simulink model "pitchAndRoll"  (R2025a)
settings: Solver=FixedStepAuto  StartTime=0.0  StopTime=30  FixedStep=0.005  RelTol=1e-3
model workspace (MAT data in the model file):
  lowerLimit = 25
  speedMax = 10
  upperLimit = 75
libraries: simulink x3, simulink_extras x1
settings Model: PacingRate=0.100000  ParameterArgumentNames=speedMax  LastModifiedBy=alexc
settings SolverCC: ZeroCrossAlgorithm=Adaptive
settings OptimizationCC: BlockReduction=off  DefaultParameterBehavior=Inlined  BufferReuse=off
settings DebuggingCC: IgnoredZcDiagnostic=none
settings RTWCC: GPUComputeCapability=3.5

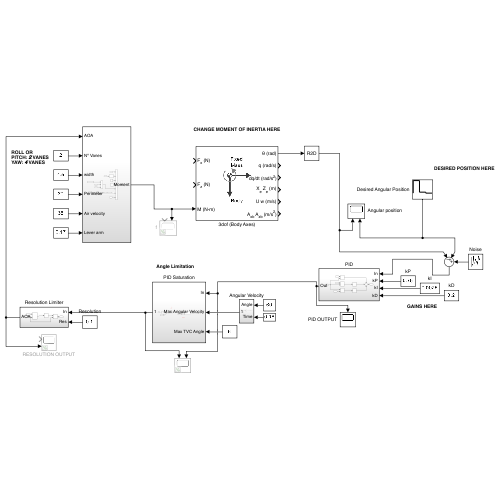
[thumbnail: Simulink's stored preview of the top-level diagram]
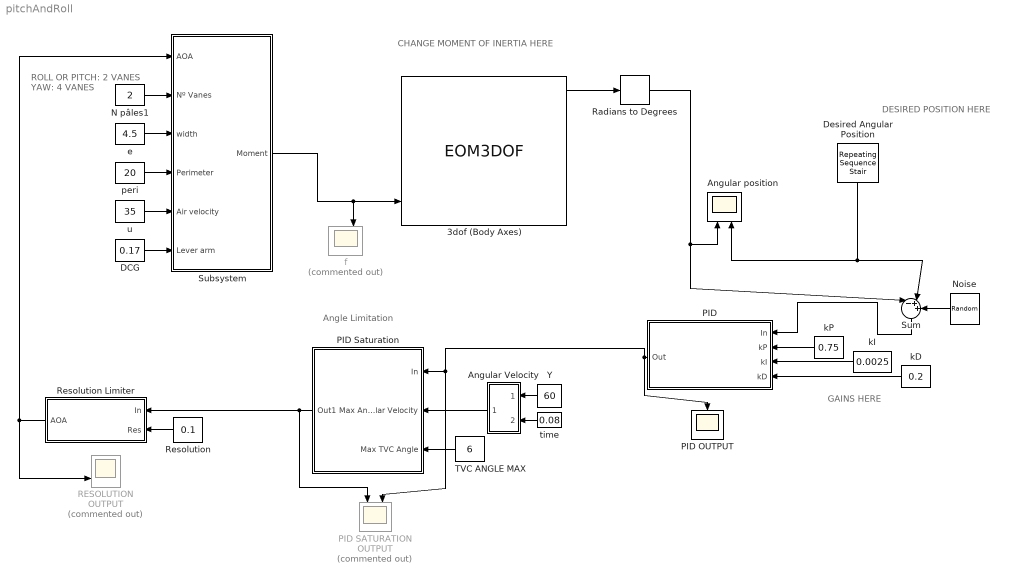
== system pitchAndRoll ==
  note: Angle Limitation
  note: GAINS HERE
  note: DESIRED POSITION HERE
  note: CHANGE MOMENT OF INERTIA HERE
  note: ROLL OR PITCH: 2 VANES
      | YAW: 4 VANES
  3dof (Body Axes) : EOM3DOF  mass=4.4  Iyy=0.045
  Angular Velocity : Subsystem
  Angular position : Scope  NumInputPorts=2
      settings: ActiveDisplayYMinimum=-1.25  ActiveDisplayYMaximum=11.25
  DCG : Constant  Value=0.17
  Desired Angular Position : simulink/Sources/Repeating Sequence Stair  OutValues=[10 2.5 2]  tsamp=1  OutMin=[]  OutMax=[]  OutDataTypeStr=double  OutputDataTypeScalingMode=double  OutDataType=fixdt(0,8)  ConRadixGroup=Best Precision: Vector-wise  OutScaling=2^-12
  N pâles1 : Constant  Value=2
  Noise : UniformRandomNumber  Minimum=-0.2  Maximum=0.2  Seed=414  SampleTime=0.02
  PID : Subsystem
  PID OUTPUT : Scope
      settings: ActiveDisplayYMinimum=-109.29716  ActiveDisplayYMaximum=117.18163  DataLoggingVariableName=ScopeData2
  PID SATURATION OUTPUT : Scope  Commented=on  NumInputPorts=2
      settings: ActiveDisplayYMinimum=-14.97719  ActiveDisplayYMaximum=15.01757  DataLoggingVariableName=ScopeData3
  PID Saturation : Subsystem
  RESOLUTION OUTPUT : Scope  Commented=on  NumInputPorts=2
      settings: ActiveDisplayYMinimum=-4.75  ActiveDisplayYMaximum=4.75
  Radians to Degrees : simulink_extras/Transformations/Radians to Degrees
  Resolution : Constant  Value=0.1
  Resolution Limiter : Subsystem
  Subsystem : Subsystem
  Sum : Sum  Inputs=|-++
  TVC ANGLE MAX : Constant  Value=6
  Y : Constant  Value=60
  e : Constant  Value=4.5
  f : Scope  Commented=on  NumInputPorts=2
      settings: ActiveDisplayYMinimum=-0.10188  ActiveDisplayYMaximum=0.10188  DataLoggingVariableName=ScopeData3
  kD : Constant  Value=0.2
  kI : Constant  Value=0.0025
  kP : Constant  Value=0.75
  peri : Constant  Value=20
  time : Constant  Value=0.08
  u : Constant  Value=35
  wires:
  Desired Angular Position/1 -> Angular position/2, Sum/2
  Radians to Degrees/1 -> Angular position/1, Sum/1
  3dof (Body Axes)/1 -> Radians to Degrees/1
  N pâles1/1 -> Subsystem/2(Nº Vanes)
  Subsystem/1(Moment) -> 3dof (Body Axes)/3, f/2
  DCG/1 -> Subsystem/6(Lever arm)
  u/1 -> Subsystem/5(Air velocity)
  e/1 -> Subsystem/3(width)
  Sum/1 -> PID/1(In)
  kP/1 -> PID/2(kP)
  kI/1 -> PID/3(kI)
  kD/1 -> PID/4(kD)
  Angular Velocity/1(Out1) -> PID Saturation/2(Max Angular Velocity)
  Y/1 -> Angular Velocity/1(Angle)
  time/1 -> Angular Velocity/2(Time)
  Resolution/1 -> Resolution Limiter/2(Res)
  PID/1(Out) -> PID OUTPUT/1, PID SATURATION OUTPUT/2, PID Saturation/1(In)
  TVC ANGLE MAX/1 -> PID Saturation/3(Max TVC Angle)
  Resolution Limiter/1(AOA) -> Subsystem/1(AOA), RESOLUTION OUTPUT/2
  PID Saturation/1(Out1) -> Resolution Limiter/1(In), PID SATURATION OUTPUT/1
  Noise/1 -> Sum/3
  peri/1 -> Subsystem/4(Perimeter)

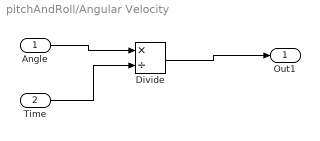
== system pitchAndRoll/Angular Velocity ==
  Angle : Inport
  Time : Inport  Port=2
  Divide : Product  Inputs=*/
  Out1 : Outport
  wires:
  Time/1 -> Divide/2
  Angle/1 -> Divide/1
  Divide/1 -> Out1/1

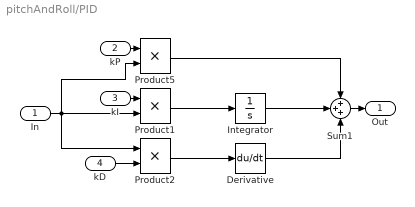
== system pitchAndRoll/PID ==
  In : Inport
  kP : Inport  Port=2
  kI : Inport  Port=3
  kD : Inport  Port=4
  Derivative : Derivative
  Integrator : Integrator
  Product1 : Product
  Product2 : Product
  Product5 : Product
  Sum1 : Sum  Inputs=+++
  Out : Outport
  wires:
  Product1/1 -> Integrator/1
  kD/1 -> Product2/2
  kI/1 -> Product1/1
  kP/1 -> Product5/1
  In/1 -> Product5/2, Product1/2, Product2/1
  Product2/1 -> Derivative/1
  Derivative/1 -> Sum1/3
  Integrator/1 -> Sum1/2
  Product5/1 -> Sum1/1
  Sum1/1 -> Out/1

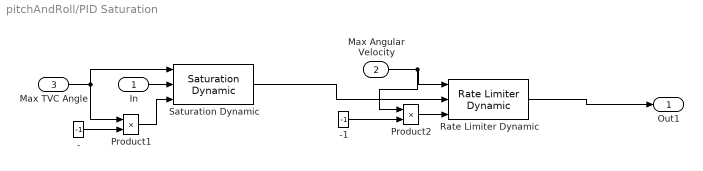
== system pitchAndRoll/PID Saturation ==
  In : Inport
  Max Angular Velocity : Inport  Port=2
  Max TVC Angle : Inport  Port=3
  - : Constant  Value=-1
  -1 : Constant  Value=-1
  Product1 : Product
  Product2 : Product
  Rate Limiter Dynamic : simulink/Discontinuities/Rate Limiter Dynamic
  Saturation Dynamic : simulink/Discontinuities/Saturation Dynamic  OutMin=[]  OutMax=[]  OutDataTypeStr=Inherit: Same as second input  OutDataType=fixdt(1, 16)  OutScaling=2^-10  DoSatur=off
  Out1 : Outport
  wires:
  Max TVC Angle/1 -> Saturation Dynamic/1, Product1/1
  -/1 -> Product1/2
  In/1 -> Saturation Dynamic/2
  Product1/1 -> Saturation Dynamic/3
  Saturation Dynamic/1 -> Rate Limiter Dynamic/2
  ? -> ?
  Max Angular Velocity/1 -> Product2/1, Rate Limiter Dynamic/1
  -1/1 -> Product2/2
  Product2/1 -> Rate Limiter Dynamic/3
  ? -> ?
  Rate Limiter Dynamic/1 -> Out1/1

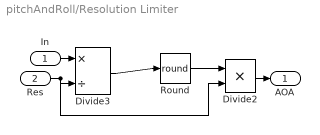
== system pitchAndRoll/Resolution Limiter ==
  In : Inport
  Res : Inport  Port=2
  Divide2 : Product  Inputs=**
  Divide3 : Product  Inputs=*/
  Round : Rounding  Operator=round
  AOA : Outport
  wires:
  In/1 -> Divide3/1
  Res/1 -> Divide2/2, Divide3/2
  Divide3/1 -> Round/1
  Round/1 -> Divide2/1
  Divide2/1 -> AOA/1

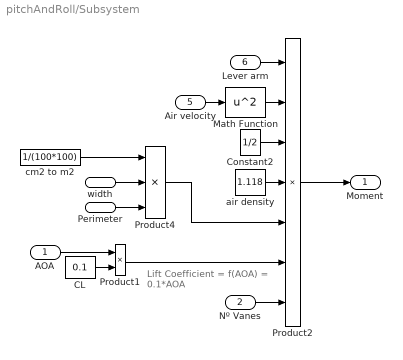
== system pitchAndRoll/Subsystem ==
  note: Lift Coefficient = f(AOA) = 0.1*AOA
  AOA : Inport
  Nº Vanes : Inport  Port=2
  width : Inport  Port=3
  Perimeter : Inport  Port=4
  Air velocity : Inport  Port=5
  Lever arm : Inport  Port=6
  CL : Constant  Value=0.1
  Constant2 : Constant  Value=1/2
  Math Function : Math  Operator=square
  Product1 : Product
  Product2 : Product  Inputs=7
  Product4 : Product  Inputs=3
  air density : Constant  Value=1.118
  cm2 to m2 : Constant  Value=1/(100*100)
  Moment : Outport
  wires:
  Math Function/1 -> Product2/2
  air density/1 -> Product2/4
  width/1 -> Product4/2
  Air velocity/1 -> Math Function/1
  Product4/1 -> Product2/5
  cm2 to m2/1 -> Product4/1
  Constant2/1 -> Product2/3
  Product2/1 -> Moment/1
  CL/1 -> Product1/2
  AOA/1 -> Product1/1
  Perimeter/1 -> Product4/3
  Nº Vanes/1 -> Product2/7
  Lever arm/1 -> Product2/1
  Product1/1 -> Product2/6
